simulink model "Receive_Ethernet_UDP - Copy"  (R2024a)
settings: Solver=ode4  StartTime=0.0  StopTime=inf  FixedStep=0.01  RelTol=1e-3
undefined symbols (not defined in the file or in its folder): f, gray
libraries: dspnetwork x1, sldrtlib x1, instrumentlib x1
settings Model: Creator=hyeon-yongjeong  LastModifiedBy=LG gram 17 - HW dev
settings HardwareCC: ProdBitPerLong=64  ProdHWDeviceType=Intel->x86-64 (Linux 64)
settings SFSimCC: SimTargetLang=C++
settings RTWCC: Description=Simulink Desktop Real-Time  SystemTargetFile=sldrt.tlc  TemplateMakefile=sldrt.tmf  TargetLang=C++  RTWCompilerOptimization=on
settings CodeAppCC: MaxIdLength=95
settings SimulinkDesktopRealTimeCC: TargetLibSuffix=_sldrt.a  TargetPreCompLibLocation=C:\Program Files\MATLAB\R2024a\toolbox\sldrt\lib\win64  TargetLangStandard=C++11 (ISO)

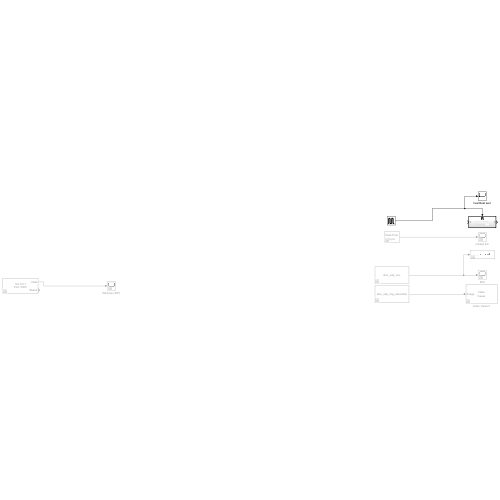
[thumbnail: Simulink's stored preview of the top-level diagram]
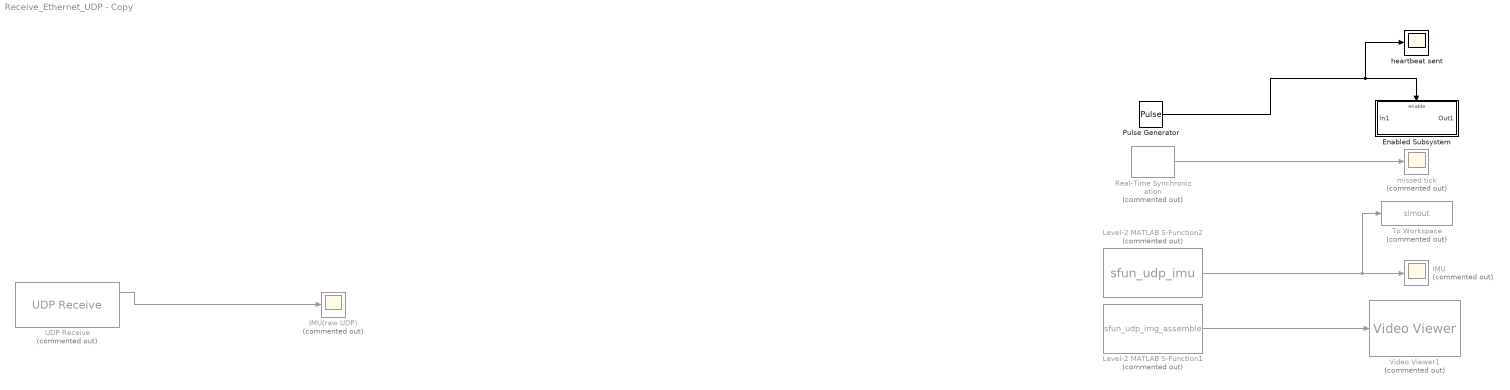
== system Receive_Ethernet_UDP - Copy ==
  Enabled Subsystem : Subsystem  TreatAsAtomicUnit=on
  IMU : Scope  Commented=on
  IMU(raw UDP) : Scope  Commented=on
  Level-2 MATLAB S-Function1 : M-S-Function  Commented=on  FunctionName=sfun_udp_img_assemble  Parameters=5006, [240 320], 10000, 0.1
  Level-2 MATLAB S-Function2 : M-S-Function  Commented=on  FunctionName=sfun_udp_imu  Parameters=5005, 0.01
  Pulse Generator : DiscretePulseGenerator  PulseType=Time based  Period=2*0.01  PulseWidth=50
  Real-Time Synchronization : sldrtlib/Real-Time Synchronization  Commented=on  SampleTime=0.01  MaxMissedTicks=inf  ShowMissedTicks=on  YieldWhenWaiting=off
  To Workspace : ToWorkspace  Commented=on  VariableName=simout  SaveFormat=Timeseries  SampleTime=-1
  UDP Receive : instrumentlib/UDP Receive  Commented=on  LocalAddress=127.0.0.1  LocalPort=5005  EnablePortSharing=off  Host=0.0.0.0  Port=5005  GetLatestData=off  DataSize=[6 1]  DataType=single  ASCIIFormatting=%f,  Terminator=LF  CustomTerminator=10  ByteOrder=little-endian  EnableBlockingMode=off  Timeout=10  SampleTime=0.01  SimulateUsing=Interpreted execution
  Video Viewer1 : VideoViewer  Commented=on  colormapValue=gray(256)  FigPos=[2873 1626.66666666667 652 454]
  heartbeat sent : Scope
  missed tick : Scope  Commented=on
  wires:
  UDP Receive/1 -> IMU(raw UDP)/1
  Level-2 MATLAB S-Function1/1 -> Video Viewer1/1
  Real-Time Synchronization/1 -> missed tick/1
  Level-2 MATLAB S-Function2/1 -> IMU/1, To Workspace/1
  Pulse Generator/1 -> heartbeat sent/1, Enabled Subsystem/Enable

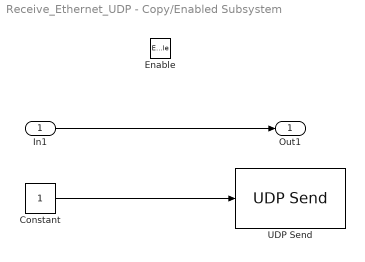
== system Receive_Ethernet_UDP - Copy/Enabled Subsystem ==
  In1 : Inport
  Enable : EnablePort
  Constant : Constant
  UDP Send : dspnetwork/UDP Send  remoteURL='127.0.0.1'  remotePort=6000  localURL='0.0.0.0'  localPortSource=Automatically determine  localPort=-1  sendBufferSize=8192  sampletime=-1  blockPlatform=HOST  separateLengthPort=0
      settings: LibrarySourceBlock=embeddedtargetslib/Host Communication/UDP Send
  Out1 : Outport
  wires:
  In1/1 -> Out1/1
  Constant/1 -> UDP Send/1
